simulink model "progetto"  (R2023b)
settings: Solver=VariableStepAuto  StartTime=0.0  StopTime=10.0  RelTol=1e-3
settings Model: Creator=Windows  LastModifiedBy=gianvincenzoconcia
settings SolverCC: AlgebraicLoopSolver=TrustRegion
settings DebuggingCC: UnconnectedInputMsg=warning  UnconnectedOutputMsg=warning  UnconnectedLineMsg=warning
settings ModelReferenceCC: EnableRefExpFcnMdlSchedulingChecks=on
settings RTWCC: DLArmComputeVersion=19.05

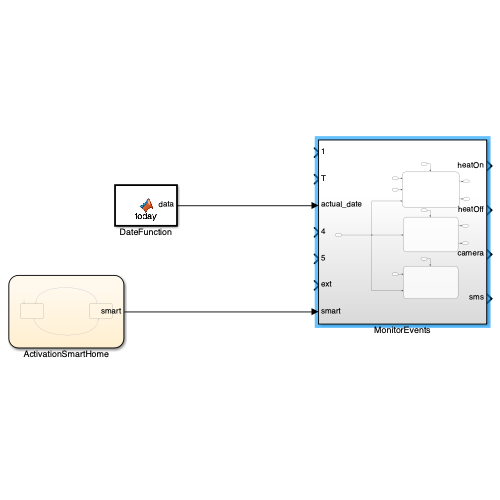
[thumbnail: Simulink's stored preview of the top-level diagram]
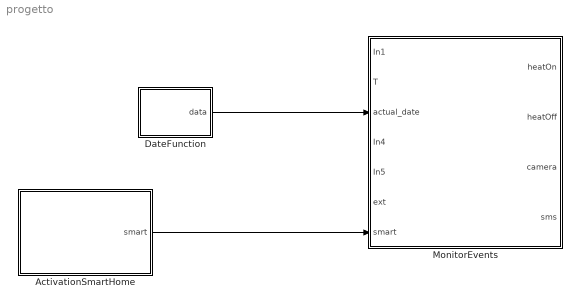
== system progetto ==
  ActivationSmartHome : Stateflow chart  TreatAsAtomicUnit=on
  DateFunction : MATLAB Function  TreatAsAtomicUnit=on
  MonitorEvents : Subsystem
  wires:
  ActivationSmartHome/1(smart) -> MonitorEvents/7(smart)
  DateFunction/1(data) -> MonitorEvents/3(actual_date)

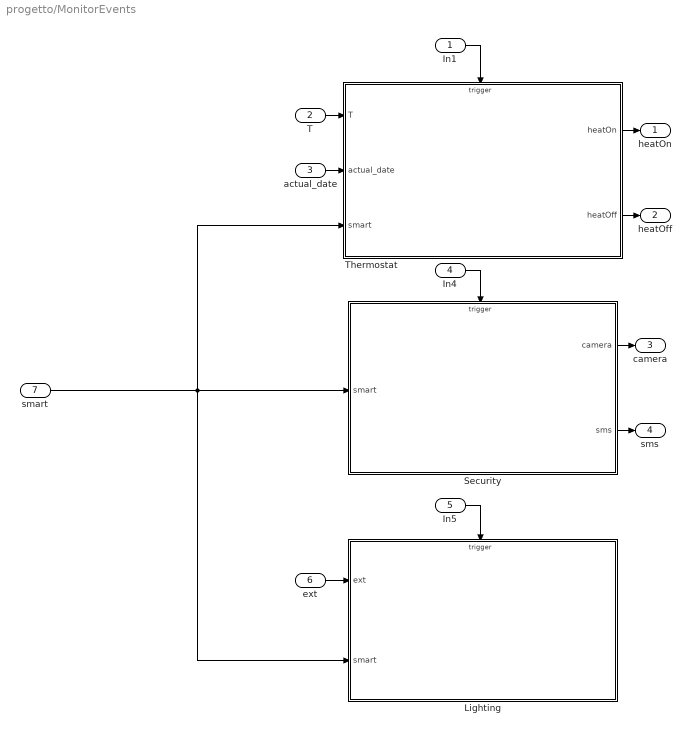
== system progetto/MonitorEvents ==
  In1 : Inport
  T : Inport  Port=2
  actual_date : Inport  Port=3
  In4 : Inport  Port=4
  In5 : Inport  Port=5
  ext : Inport  Port=6
  smart : Inport  Port=7
  Lighting : Stateflow chart  TreatAsAtomicUnit=on
  Security : Stateflow chart  TreatAsAtomicUnit=on
  Thermostat : Stateflow chart  TreatAsAtomicUnit=on
  heatOn : Outport
  heatOff : Outport  Port=2
  camera : Outport  Port=3
  sms : Outport  Port=4
  wires:
  In4/1 -> Security/Trigger
  Security/1(camera) -> camera/1
  Thermostat/2(heatOff) -> heatOff/1
  In5/1 -> Lighting/Trigger
  T/1 -> Thermostat/1(T)
  In1/1 -> Thermostat/Trigger
  ext/1 -> Lighting/1(ext)
  Security/2(sms) -> sms/1
  actual_date/1 -> Thermostat/2(actual_date)
  Thermostat/1(heatOn) -> heatOn/1
  smart/1 -> Thermostat/3(smart), Lighting/2(smart), Security/1(smart)

== matlab function progetto/DateFunction ==
  data: data output
function data = today()
    today = datetime("now");
    data = month(today) + "-" + year(today);
end

== stateflow chart progetto/ActivationSmartHome ==
  state Inattivo
    en:
    smart == 0;
  state Attivo
    du:
    smart == 1;
  Attivo -> Inattivo : user_exit
  (default) -> Inattivo
  Inattivo -> Attivo : user_entry
  data: smart output

== stateflow chart progetto/MonitorEvents/Lighting ==
  state Light_on
    en:
    light = true;
    state Increment_int_light
      du:
      ext = ext - 1;
      int = int + 1;
    state Decrement_int_light
      du:
      ext = ext + 1;
      int = int - 1;
    (default) -> Increment_int_light
    Decrement_int_light -> Increment_int_light : [ext == 10 && int == 1]
    Increment_int_light -> Decrement_int_light : [ext == 1 && int == 10]
  state Light_off
    en:
    light = false;
  (default) -> Light_on
  Light_on -> Light_off : [smart == 0 && user_off]
  Light_off -> Light_on : [smart == 1 && user_on]
  data: ext input; smart input
  events: user_off input RISING_EDGE_EVENT; user_on input RISING_EDGE_EVENT

== stateflow chart progetto/MonitorEvents/Security ==
  state Antitheft
    state Idle
      en:
      camera = 0;
      sms = 0;
    state Armed
      du:
      camera = 1;
    state Alarm
      du:
      camera = 1;
      sms = 1;
    (default) -> Idle
    Idle -> Armed : [smart == 0]{camera = 1}
    Armed -> Idle [order 2] : [smart == 1]{camera = 0}
    Alarm -> Idle : [user_off]{camera = 0}
    Armed -> Alarm [order 1] : [intrusion]{sms = 1}
  (default) -> Antitheft
  data: camera output; sms output; smart input
  events: intrusion input RISING_EDGE_EVENT

== stateflow chart progetto/MonitorEvents/Thermostat ==
  state Thermostat
    state ON
      en: thermos == 1;
      state heating
      state cooling
      (default) -> heating
      heating -> cooling : [T >= 22]{heatOn}
      cooling -> heating : [T < 17]{heatOff}
    state OFF
      en: thermos == 0;
    ON -> OFF : [stop]
    OFF -> ON : [start]
    (default) -> OFF
  state Season
    en:
    cooling_date = datetime('01-Oct', 'Format', 'dd-MMM');
    heating_date = datetime('01-Apr', 'Format', 'dd-MMM');
    state hot
    state cold
    (default) -> hot
    hot -> cold : [smart == 1 && actual_date > cooling_date && actual_date < heating_date]{send(start, Thermostat)}
    cold -> hot : [smart == 0 || actual_date < cooling_date && actual_date > heating_date]{send(stop, Thermostat)}
  (default) -> Season
  data: T input; heatOn output; heatOff output; actual_date input; cooling_date constant double; heating_date constant double; smart input
  events: start input RISING_EDGE_EVENT; stop input RISING_EDGE_EVENT
